simulink model "hw4q3a"  (R2019b)
settings: Solver=FixedStepAuto  StartTime=0.0  StopTime=20  FixedStep=0.01  RelTol=1e-3
libraries: slident x2
settings Model: Creator=axs2437  LastModifiedBy=axs2437
settings DataIOCC: ReturnWorkspaceOutputs=off

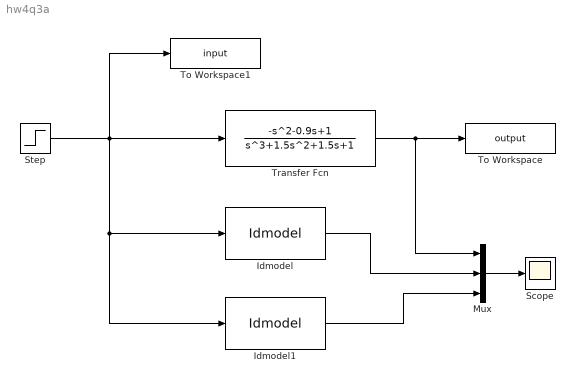
== system hw4q3a ==
  Idmodel : slident/Models/Idmodel  sys=ContinuousSS4  IC=0  noi=off  seed=[]
      settings: SourceProductName=System Identification Toolbox  SourceProductBaseCode=ID
  Idmodel1 : slident/Models/Idmodel  sys=DiscreteSS4  IC=0  noi=off  seed=[]
      settings: SourceProductName=System Identification Toolbox  SourceProductBaseCode=ID
  Mux : Mux  Inputs=3
  Scope : Scope
  Step : Step  SampleTime=0.01
  To Workspace : ToWorkspace  VariableName=output  SampleTime=-1
  To Workspace1 : ToWorkspace  VariableName=input  SampleTime=-1
  Transfer Fcn : TransferFcn  Numerator=[-1 -0.9 1]  Denominator=[1 1.5 1.5 1]
  wires:
  Step/1 -> Idmodel1/1, Idmodel/1, Transfer Fcn/1, To Workspace1/1
  Transfer Fcn/1 -> Mux/1, To Workspace/1
  Idmodel/1 -> Mux/2
  Idmodel1/1 -> Mux/3
  Mux/1 -> Scope/1
